simulink model "ModelSimpleSrc"  (R2022b)
settings: Solver=FixedStepDiscrete  StartTime=0.0  StopTime=1.0  RelTol=1e-3  EnableMultiTasking=on
InitFcn:
  | ModelSimpleSrcSettings=BTConfig.GetModelSettings();
  | 
  | ModelSimpleSrcSettings.Validate();
  | ModelSimpleSrcSettings.DoMaskInit('ModelSimpleSrcSettings');
libraries: EdgePorts x6, HandyTextFile x2, dspsrcs4 x2, SampleRateConverterBtc x2, FeaturePath x1
settings Model: Creator=kl13806  LastModifiedBy=sc48041
settings OptimizationCC: DefaultParameterBehavior=Inlined  EnhancedBackFolding=on  ZeroExternalMemoryAtStartup=off  ZeroInternalMemoryAtStartup=off  OptimizeBlockOrder=speed  DifferentSizesBufferReuse=on  OptimizationCustomize=off  EfficientTunableParamExpr=on
settings DebuggingCC: MultiTaskDSMMsg=none  ParameterTunabilityLossMsg=error
settings HardwareCC: TargetBitPerPointer=64  TargetBitPerSizeT=64  TargetBitPerPtrDiffT=64  TargetLongLongMode=on  TargetIntDivRoundTo=Zero  TargetEndianess=LittleEndian  TargetWordSize=64  TargetHWDeviceType=MATLAB Host  ProdEqTarget=off
settings ModelReferenceCC: ModelReferenceNumInstancesAllowed=Single
settings SFSimCC: MATLABDynamicMemAlloc=off
settings RTWCC: Description=Embedded Coder (host-based shared library target)  SystemTargetFile=ert_shrlib.tlc  GenCodeOnly=on  TemplateMakefile=ert_default_tmf
settings CodeAppCC: ForceParamTrailComments=on  IgnoreCustomStorageClasses=off  OperatorAnnotations=on  SimulinkDataObjDesc=on  SFDataObjDesc=on  InsertBlockDesc=on
settings STFCustomTargetCC: TargetLangStandard=C99 (ISO)  MultiwordLength=256  GenerateSampleERTMain=on  ParMdlRefBuildCompliant=on  CompOptLevelCompliant=on  CombineOutputUpdateFcns=on  ERTCustomFileBanners=on  SupportContinuousTime=off  SupportNonInlinedSFcns=off  RemoveResetFunc=on  MATLABClassNameForMDSCustomization=Simulink.SoftwareTarget.ERTCustomization  ModelStepFunctionPrototypeControlCompliant=on  UseToolchainInfoCompliant=on  SystemTargetFile=ert_shrlib.tlc
settings ERTTargetCC: TargetLangStandard=C99 (ISO)  GenerateSampleERTMain=on  ConcurrentExecutionCompliant=off  CPPClassGenCompliant=off  InlinedParameterPlacement=NonHierarchical  ERTSrcFileBannerTemplate=bose_ert_code_template.cgt  ERTHdrFileBannerTemplate=bose_ert_code_template.cgt  ERTDataSrcFileTemplate=bose_ert_code_template.cgt  ERTDataHdrFileTemplate=bose_ert_code_template.cgt  ERTCustomFileTemplate=example_file_process.tlc

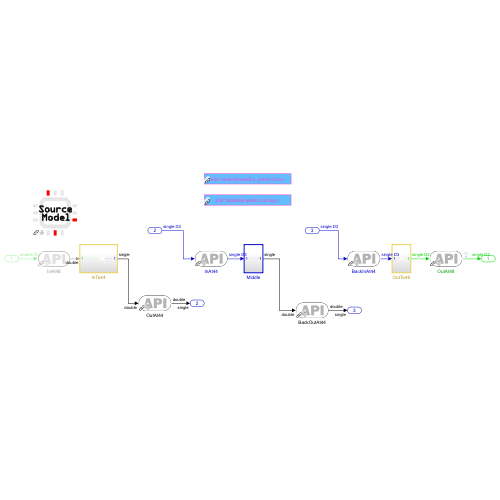
[thumbnail: Simulink's stored preview of the top-level diagram]
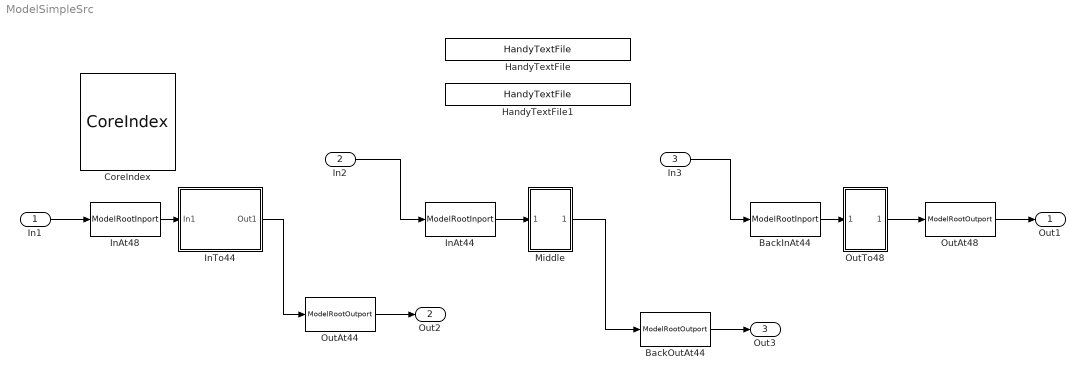
== system ModelSimpleSrc ==
  In1 : Inport
  In2 : Inport  Port=2
  In3 : Inport  Port=3
  BackInAt44 : EdgePorts/ModelRootInport  Config=ModelSimpleSrcSettings.BackInAt44
      settings: SourceProductName=Bose Talaria
  BackOutAt44 : EdgePorts/ModelRootOutport  Config=ModelSimpleSrcSettings.BackOutAt44
      settings: SourceProductName=Bose Talaria
  CoreIndex : FeaturePath/CoreIndex  Role=Source Model  CoreIndex=8  Config=ModelSimpleSrcSettings.CoreIndex  AddressingMode=Directly include core number in message identifiers (i.e. simple and static)  CrossCoreApi=FourListChipManager  CrossCoreAllocation=LocalCore  CrossCoreSampleTime=-1  BasePeriod=[]  TriggerInit=[135 64 230 161]
      settings: SourceProductName=Bose Talaria
  HandyTextFile : HandyTextFile/HandyTextFile  TemplateSource=<dialog fields>  FileSuffix=_atomicList  OpenDialogOnLoad=off  UseThisBlockName=off  AddGrandParentNamePrefix=off  TheDefaultText=% $(FILENAME) $(PREFIX) $(SUFFIX)  ShowInLibBrowser=on
      settings: SourceProductName=Bose Talaria
  HandyTextFile1 : HandyTextFile/HandyTextFile  TemplateSource=<dialog fields>  FileSuffix=Config  OpenDialogOnLoad=off  UseThisBlockName=off  AddGrandParentNamePrefix=off  TheDefaultText=% $(FILENAME) $(PREFIX) $(SUFFIX)  ShowInLibBrowser=on
      settings: SourceProductName=Bose Talaria
  InAt44 : EdgePorts/ModelRootInport  Config=ModelSimpleSrcSettings.InAt44
      settings: SourceProductName=Bose Talaria
  InAt48 : EdgePorts/ModelRootInport  Config=ModelSimpleSrcSettings.InAt48
      settings: SourceProductName=Bose Talaria
  InTo44 : Subsystem  TreatAsAtomicUnit=on
  Middle : Subsystem  TreatAsAtomicUnit=on
  OutAt44 : EdgePorts/ModelRootOutport  Config=ModelSimpleSrcSettings.OutAt44
      settings: SourceProductName=Bose Talaria
  OutAt48 : EdgePorts/ModelRootOutport  Config=ModelSimpleSrcSettings.OutAt48
      settings: SourceProductName=Bose Talaria
  OutTo48 : Subsystem  TreatAsAtomicUnit=on
  Out1 : Outport
  Out2 : Outport  Port=2
  Out3 : Outport  Port=3
  wires:
  In1/1 -> InAt48/1
  OutAt48/1 -> Out1/1
  OutTo48/1(Out1) -> OutAt48/1
  InAt48/1 -> InTo44/1(In1)
  InAt44/1 -> Middle/1(In1)
  In2/1 -> InAt44/1
  BackInAt44/1 -> OutTo48/1(In1)
  In3/1 -> BackInAt44/1
  OutAt44/1 -> Out2/1
  InTo44/1(Out1) -> OutAt44/1
  BackOutAt44/1 -> Out3/1
  Middle/1(Out1) -> BackOutAt44/1

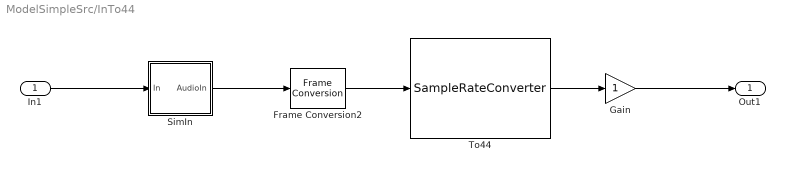
== system ModelSimpleSrc/InTo44 ==
  In1 : Inport  SampleTime=32/48000
  Frame Conversion2 : FrameConversion
  Gain : Gain
  SimIn : Subsystem  TreatAsAtomicUnit=on
  To44 : SampleRateConverterBtc/SampleRateConverter  Config=ModelSimpleSrcSettings.To44
      settings: SourceProductName=Bose Blocklib
  Out1 : Outport
  wires:
  Gain/1 -> Out1/1
  To44/1 -> Gain/1
  Frame Conversion2/1 -> To44/1
  In1/1 -> SimIn/1(In)
  SimIn/1(AudioIn) -> Frame Conversion2/1

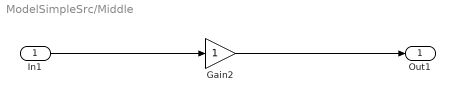
== system ModelSimpleSrc/Middle ==
  In1 : Inport
  Gain2 : Gain
  Out1 : Outport
  wires:
  In1/1 -> Gain2/1
  Gain2/1 -> Out1/1

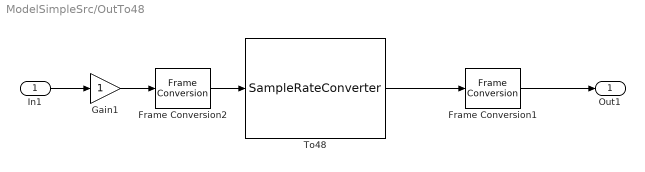
== system ModelSimpleSrc/OutTo48 ==
  In1 : Inport
  Frame Conversion1 : FrameConversion  OutFrame=Sample-based
  Frame Conversion2 : FrameConversion
  Gain1 : Gain
  To48 : SampleRateConverterBtc/SampleRateConverter  Config=ModelSimpleSrcSettings.To48
      settings: SourceProductName=Bose Blocklib
  Out1 : Outport
  wires:
  To48/1 -> Frame Conversion1/1
  Gain1/1 -> Frame Conversion2/1
  In1/1 -> Gain1/1
  Frame Conversion1/1 -> Out1/1
  Frame Conversion2/1 -> To48/1

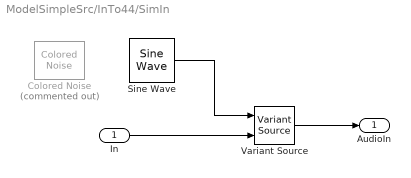
== system ModelSimpleSrc/InTo44/SimIn ==
  In : Inport  OutDataTypeStr=single  SampleTime=32/48000
  Colored Noise : dspsrcs4/Colored Noise  Commented=on  Color=pink  InverseFrequencyPower=1  BoundedOutput=on  NumChannels=2  OutputDataType=single  SamplesPerFrame=32  SampleTime=1/48000  RandomStream=mt19937ar with seed  Seed=67  SimulateUsing=Interpreted execution
  Sine Wave : dspsrcs4/Sine Wave  Amplitude=[ones(1,5)]  Frequency=[150 225 300 325 375]  Phase=zeros(1,5)  SampleMode=Discrete  OutComplex=Real  CompMethod=Trigonometric fcn  TableSize=Speed  SampleTime=1/48000  SamplesPerFrame=32  ResetState=Restart at time zero  OutputFrames=off  dataType=single  wordLen=16  udDataType=sfix(16)  fracBitsMode=Best precision  numFracBits=15  OutDataTypeStr=single  LastOutDataTypeStr=single
  Variant Source : VariantSource  VariantControlMode=sim codegen switching  ShowConditionOnBlock=on
  AudioIn : Outport  VectorParamsAs1DForOutWhenUnconnected=off
  wires:
  In/1 -> Variant Source/2
  Variant Source/1 -> AudioIn/1
  Sine Wave/1 -> Variant Source/1
